simulink model "sim_SoftwareIntheLoop_Compensator"  (R2018a)
settings: Solver=ode3  StartTime=0.0  StopTime=40  FixedStep=0.005  RelTol=1e-3  EnableMultiTasking=on
InitFcn:
  | % load parameters of the default quadrotor
  | disp('Quadrotor parameters loaded by InitFcn')
  | parameters_estimationcontrol %load mdl_quadcopter as well!
  | 
  | % change to Simulation folder if in data folder
  | %cd([matlabpath '/Simulation']);
values from neighbouring files (symbols this model uses):
  controlHelperParams =     [LQR_param.mat]
  estimParams =     [LQR_param.mat]
  quad =     [LQR_param.mat]
  quadEDT =     [LQR_param.mat]
undefined symbols (not defined in the file or in its folder): DiscIntNeverNeededParam, Discrete, RSrun_sensordataCalib, rt_yout, Time
libraries: simulink x25, ctrlSharedLib x3
(part 2 of 2)

== matlab function sim_SoftwareIntheLoop_Compensator/Drone_Compensator/Estimator/EstimatorXYPosition/EstimatorVelocity/AccelerationHandling/trafo_World2Body_trans ==
  data: orientation input; vector input; y output
function y = fcn(orientation,vector)

yaw     = orientation(1);
pitch   = orientation(2);
roll    = orientation(3);

R_World2Body = [[                                cos(pitch)*cos(yaw),                                cos(pitch)*sin(yaw),          -sin(pitch)];
                    [ cos(yaw)*sin(pitch)*sin(roll) - cos(roll)*sin(yaw), cos(roll)*cos(yaw) + sin(pitch)*sin(roll)*sin(yaw), cos(pitch)*sin(roll)];
                    [ sin(roll)*sin(yaw) + cos(roll)*cos(yaw)*sin(pitch), cos(roll)*sin(pitch)*sin(yaw) - cos(yaw)*sin(roll), cos(pitch)*cos(roll)]];

y = R_World2Body*vector;

== matlab function sim_SoftwareIntheLoop_Compensator/Drone_Compensator/Estimator/EstimatorXYPosition/EstimatorXYPosition/trafo_BodytoWorld_trans ==
  data: orientation input; vector input; vel_world output
function vel_world = fcn(orientation,vector)
yaw   = orientation(1);
pitch = orientation(2);
roll  = orientation(3);

R_BodytoWorld = [cos(pitch)*cos(yaw) sin(roll)*sin(pitch)*cos(yaw)-cos(roll)*sin(yaw) cos(roll)*sin(pitch)*cos(yaw)+sin(roll)*sin(yaw);   %BBF > Inertial rotation matrix
  cos(pitch)*sin(yaw) sin(roll)*sin(pitch)*sin(yaw)+cos(roll)*cos(yaw) cos(roll)*sin(pitch)*sin(yaw)-sin(roll)*cos(yaw);
  -sin(pitch)         sin(roll)*cos(pitch)                            cos(roll)*cos(pitch)];

vel_world = R_BodytoWorld*vector;

== matlab function sim_SoftwareIntheLoop_Compensator/Drone_Compensator/Estimator/EstimatorAltitude/trafo_BodytoWorld_trans ==
  data: orientation input; vector input; acc_world output
function acc_world = fcn(orientation,vector)
yaw     = orientation(1);
pitch   = orientation(2);
roll    = orientation(3);

R_BodytoWorld = [cos(pitch)*cos(yaw) sin(roll)*sin(pitch)*cos(yaw)-cos(roll)*sin(yaw) cos(roll)*sin(pitch)*cos(yaw)+sin(roll)*sin(yaw);   %BBF > Inertial rotation matrix
  cos(pitch)*sin(yaw) sin(roll)*sin(pitch)*sin(yaw)+cos(roll)*cos(yaw) cos(roll)*sin(pitch)*sin(yaw)-sin(roll)*cos(yaw);
  -sin(pitch)         sin(roll)*cos(pitch)                            cos(roll)*cos(pitch)];

acc_world = R_BodytoWorld*vector;

== matlab function sim_SoftwareIntheLoop_Compensator/Drone_Compensator/Estimator/EstimatorAltitude/trafo_WorldToBody_trans ==
  data: orientation input; vector input; acc_RS output
function acc_RS = fcn(orientation,vector)
yaw     = orientation(1);
pitch   = orientation(2);
roll    = orientation(3);


R_World2Body = [[                                cos(pitch)*cos(yaw),                                cos(pitch)*sin(yaw),          -sin(pitch)];
                    [ cos(yaw)*sin(pitch)*sin(roll) - cos(roll)*sin(yaw), cos(roll)*cos(yaw) + sin(pitch)*sin(roll)*sin(yaw), cos(pitch)*sin(roll)];
                    [ sin(roll)*sin(yaw) + cos(roll)*cos(yaw)*sin(pitch), cos(roll)*sin(pitch)*sin(yaw) - cos(yaw)*sin(roll), cos(pitch)*cos(roll)]];

acc_RS = R_World2Body*vector;

== matlab function sim_SoftwareIntheLoop_Compensator/Drone_Compensator/Estimator/EstimatorOrientation ==
  data: sensorIMU_datin input; yawVIS_datin input; validVIS_flagin input; g input; orient_estimout output; dt input; dorient_estimout output; deuler_datout output; imuAbs_datout output
function [orient_estimout, dorient_estimout,deuler_datout,imuAbs_datout]  = fcn(sensorIMU_datin, yawVIS_datin, validVIS_flagin, g, dt)
persistent yaw_cur pitch_cur roll_cur

p = sensorIMU_datin(4);
q = sensorIMU_datin(5);
r = sensorIMU_datin(6);

if isempty(yaw_cur)
   yaw_cur = 0;
end
if isempty(pitch_cur)
   pitch_cur = 0;
end
if isempty(roll_cur)
   roll_cur = 0;
end

[yaw,pitch,roll,deuler_datout,imuAbs_datout]= complimentaryfilter(yaw_cur, pitch_cur, roll_cur, g, dt,sensorIMU_datin, yawVIS_datin,validVIS_flagin);

yaw_cur     = yaw;
pitch_cur   = pitch;
roll_cur    = roll;

orient_estimout     = [yaw,pitch,roll]';
dorient_estimout    = [p,q,r]';

== matlab function sim_SoftwareIntheLoop_Compensator/Drone_Compensator/Estimator/EstimatorXYPosition/EstimatorXYPosition/OutlierHandling/abs ==
  data: vec input; y output
function y = fcn(vec)
y = norm(vec,2);
